simulink model "voltage_droop_01"  (R2020b)
settings: Solver=VariableStepAuto  StartTime=0.0  StopTime=1  RelTol=1e-3
undefined symbols (not defined in the file): droop1
libraries: fl_lib x8, nesl_utility x4, simulink x1, aerolibanimutils x1
settings Model: Creator=gdudgeon  LastModifiedBy=gdudgeon

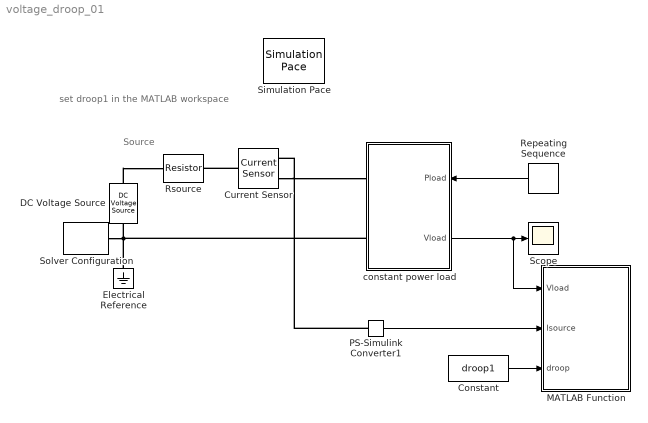
== system voltage_droop_01 ==
  note: set droop1 in the MATLAB workspace
  note: Source
  Constant : Constant  Value=droop1
  Current Sensor : fl_lib/Electrical/Electrical Sensors/Current Sensor
  DC Voltage Source : fl_lib/Electrical/Electrical Sources/DC Voltage Source  v0=1 V
      settings: AttributesFormatString=%<v0>
  Electrical Reference : fl_lib/Electrical/Electrical Elements/Electrical Reference
  MATLAB Function : MATLAB Function  TreatAsAtomicUnit=on  SystemSampleTime=Tanim  mask(Machine Rotor Animation){Tanim=0.01}
      mask prompts: Tanim "Animation Rate [s]"
      mask help: This block animates permanent magnet inside a stator. The "thetaRotor" input is the angle of the rotor. The "phase" parameter must be defined in the workspace and selects the energized coil in the stator.
  PS-Simulink Converter1 : nesl_utility/PS-Simulink Converter  PhysicalDomain=network_engine_domain  SubClassName=ps_output  LeftPortType=input  RightPortType=output  PseudoPeriodic=off  Frequencies=[]  Unit=inherit  AffineConversion=off
  Repeating Sequence : simulink/Sources/Repeating Sequence  rep_seq_t=[0 1 2]  rep_seq_y=[1e-3 1 1]
  Rsource : fl_lib/Electrical/Electrical Elements/Resistor  R=droop1*(1-droop1) Ohm  i_specify=off  i_priority=None  i=0 A  i_nominal_specify=off  i_nominal_unit=A  i_nominal_value=1  v_specify=off  v_priority=None  v=0 V  v_nominal_specify=off  v_nominal_unit=V  v_nominal_value=1
  Scope : Scope
  Simulation Pace : aerolibanimutils/Simulation Pace  SimulationPace=0.1  SleepMode=Auto  OutputPaceError=off  SampleTime=0.0001
  Solver Configuration : nesl_utility/Solver Configuration  PhysicalDomain=network_engine_domain  SubClassName=solver  LeftPortType=input  RightPortType=generic  Tones=[]  Harmonics=[]  SimulateNoise=off  Profile=off  UseLocalSampling=off  EnableSwitchedLinearOptims=on  FrequencyDomain=off  UseCCode=off  RelTol=0.001  AbsTol=1e-06  MinStep=1e-09  ToWorkspace=off  RevertToSquareIcSolve=off  NumHomotopyIterations=100  PhasorMode=off  PhasorModeNumHarmonics=1  DoDC=off  ResidualTolerance=1e-09  UseLocalSolver=on  LocalSolverChoice=NE_BACKWARD_EULER_ADVANCER  LocalSolverSampleTime=0.001  DoFixedCost=on  MaxNonlinIter=3  MaxModeIter=2  ComputeImpulses=off  ImpulseIterations=2  LinearAlgebra=auto  EquationFormulation=NE_TIME_EF  DelaysMemoryBudget=1024  AutomaticFiltering=on  FilteringTimeConstant=0.001  PartitionStorageMethod=AS_NEEDED  PartitionMemoryBudget=1024  PartitionMethod=ROBUST
  constant power load : Subsystem
      settings: PortSchema="{\"entries\":[{\"content\":{\"sides\":[{\"content\":{\"connectorIds\":[\"LConn1\",\"LConn2\"]},\"type\":\"ConnectorPlacement.EquallySpacedRectSide\",\"uuid\":\"ede3b789-4807-48db-8c98-272deebb1f90\"},{\"content\":{\"connectorIds\":[\"In1\",\"Out1\"],\"side\":\"RIGHT\"},\"type\":\"ConnectorPlacement.EquallySpacedRectSide\",\"uuid\":\"cedec5e8-adcb-43e2-ab37-681d5d79ce2a\"},{\"content\":{\"connectorIds\":[],\"side\":\"TOP\"},\"type\":\"ConnectorPlacement.EquallySpacedRectSide\",\"uuid\":\"08b52c53-b13a-4cd2-b8db-308d9ebd4277\"},{\"content\":{\"connectorIds\":[],\"side\":\"HIDDEN\"},\"type\":\"ConnectorPlacement.EquallySpacedRectSide\",\"uuid\":\"3f956204-c540-4879-b053-0f78777aeccb\"}]},\"type\":\"ConnectorPlacement.EquallySpacedConnector\",\"uuid\":\"42303a72-b7ff-4a69-b636-ebca1dcca68c\"}],\"packageUris\":[\"http://schema.mathworks.com/mf0/Connector/R2020b\"],\"version\":\"1.0\"}"
  wires:
  constant power load/1(Vload) -> MATLAB Function/1(Vload), Scope/1
  Repeating Sequence/1 -> constant power load/1(Pload)
  PS-Simulink Converter1/1 -> MATLAB Function/2(Isource)
  Constant/1 -> MATLAB Function/3(droop)
  connections:
  DC Voltage Source/LConn1 -- Rsource/LConn1
  Solver Configuration/RConn1 -- Electrical Reference/LConn1 -- constant power load/LConn2 -- DC Voltage Source/RConn1
  Current Sensor/RConn2 -- constant power load/LConn1
  Current Sensor/LConn1 -- Rsource/RConn1
  PS-Simulink Converter1/LConn1 -- Current Sensor/RConn1

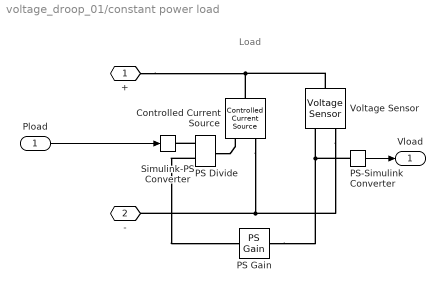
== system voltage_droop_01/constant power load ==
  note: Load
  Pload : Inport
  Controlled Current Source : fl_lib/Electrical/Electrical Sources/Controlled Current Source
  PS Divide : fl_lib/Physical Signals/Functions/PS Divide
      settings: SourceProductBaseCode=SS
  PS Gain : fl_lib/Physical Signals/Functions/PS Gain  gain=-1
  PS-Simulink Converter : nesl_utility/PS-Simulink Converter  PhysicalDomain=network_engine_domain  SubClassName=ps_output  LeftPortType=input  RightPortType=output  PseudoPeriodic=off  Frequencies=[]  Unit=inherit  AffineConversion=off
  Simulink-PS Converter : nesl_utility/Simulink-PS Converter  PhysicalDomain=network_engine_domain  SubClassName=ps_input  LeftPortType=input  RightPortType=output  PseudoPeriodic=off  Frequencies=[]  NoiseDistribution=none  NoiseParameters=[]  Unit=W  AffineConversion=off  FilteringAndDerivatives=provide  SimscapeFilterOrder=1  InputFilterTimeConstant=0.001  UdotUserProvided=0
  Voltage Sensor : fl_lib/Electrical/Electrical Sensors/Voltage Sensor
  + : PMIOPort  Side=Left
  - : PMIOPort  Port=2  Side=Left
  Vload : Outport
  wires:
  PS-Simulink Converter/1 -> Vload/1
  Pload/1 -> Simulink-PS Converter/1
  connections:
  PS-Simulink Converter/LConn1 -- PS Gain/LConn1 -- Voltage Sensor/RConn1
  PS Divide/RConn1 -- Controlled Current Source/RConn1
  Controlled Current Source/RConn2 -- Voltage Sensor/RConn2 -- -/RConn1
  PS Divide/LConn1 -- Simulink-PS Converter/RConn1
  PS Divide/LConn2 -- PS Gain/RConn1
  Voltage Sensor/LConn1 -- +/RConn1 -- Controlled Current Source/LConn1

== matlab function voltage_droop_01/MATLAB Function ==
  data: Vload input; Isource input; droop input
function plotDroop(Vload,Isource,droop)

persistent hp hp2 hf


if isempty(hf)
    
    figure(1); clf(1); hold on;
    
    [hp,hf,hp2] = plotBackground(Vload,Isource,droop);
  
    drawnow
    
else
    
    updateAnimation(hp,hp2,Vload,Isource);

    drawnow

end

end


function [hp,hf,hp2] = plotBackground(Vload,Isource,droop)

coder.extrinsic('num2str')


hf = figure(1);hold on,grid %#ok<*DUALC>

hp = plot([0 1],[1 1]*Vload);xlabel('Power (pu)'),ylabel('Voltage (pu)')
hp2 = plot([1 1]*Isource*Vload,[0.94 Vload],'k--');

plot([0 1],[1 1-droop],'r');
title(['Droop = ',num2str(droop)])

ha = gca;

end

function  updateAnimation(hp,hp2,Vload,Isource)


set(hp,'YData',[1 1]*Vload);

set(hp2,'XData',[1 1]*Isource*Vload);
set(hp2,'YData',[0.94 Vload]);

end
